simulink model "sampleModel1878"  (R2023a)
settings: Solver=VariableStepAuto  StartTime=0.0  StopTime=10.0  RelTol=1e-3
libraries: hdlsllib x5
settings Model: Creator=user1  LastModifiedBy=user1

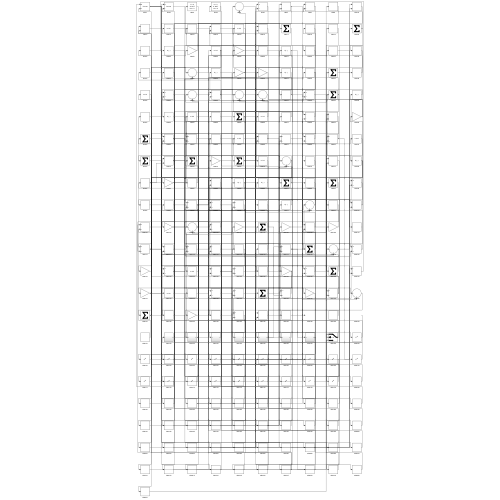
[thumbnail: Simulink's stored preview of the top-level diagram]
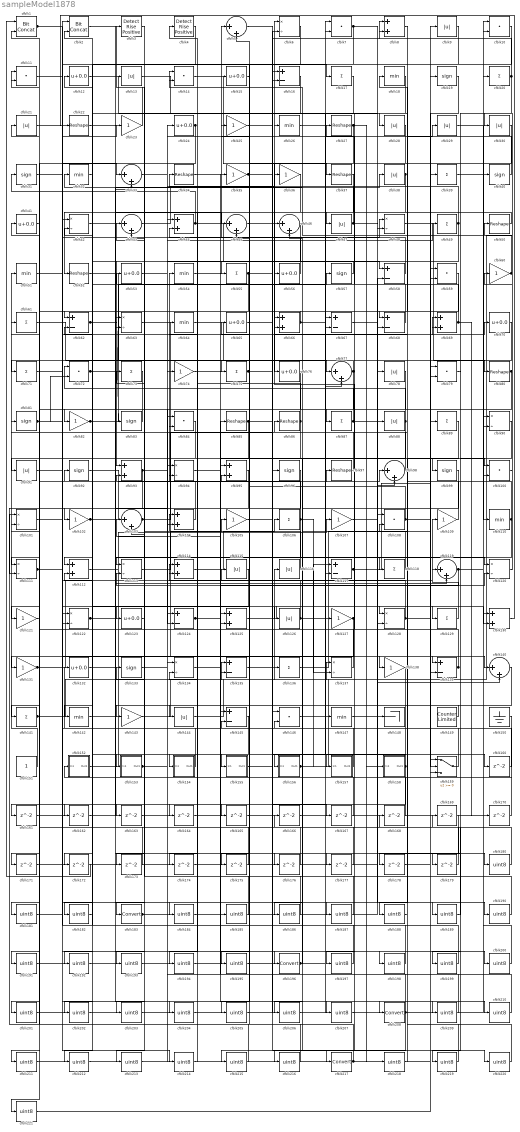
== system sampleModel1878 ==
  cfblk1 : hdlsllib/Logic and Bit Operations/Bit Concat  numInputs=2
  cfblk{7,10..11,14,59,72,79,84,100,108,146} (11 alike) : DotProduct  OutDataTypeStr=Inherit: Inherit via internal rule
  cfblk{6,42,48,63,90,94,101,111,113,120,122,128,134,137} (14 alike) : Product  Inputs=*/  RndMeth=Zero  SaturateOnIntegerOverflow=on
  cfblk{23,25,35..36,60,74,82,102,105,107,109,121,127,131,138,143} (16 alike) : Gain
  cfblk{5,33,43,45..46,77,98,103,119,140} (10 alike) : Sum  Inputs=|++
  cfblk{8,44,66,69,93,95,104,112,114,125,130} (11 alike) : Sum
  cfblk{17,20,39,49,55,61,71,73,75,87,89,106,118,129,136,141} (16 alike) : Sum  Inputs=+
  cfblk{18,26,32,51,54,64,110,142,147} (9 alike) : MinMax
  cfblk{9,13,21,28..30,38,47,78,88,91,115..116,126,144} (15 alike) : Abs  SaturateOnIntegerOverflow=off
  cfblk{16,58,62,67..68,117,124,135,139,145} (10 alike) : Sum  Inputs=+-
  cfblk{12,15,24,41,53,56,65,70,76,123,132} (11 alike) : Bias  Bias=0.0  SaturateOnIntegerOverflow=off
  cfblk{19,31,40,57,81,83,92,96,99,133} (10 alike) : Signum
  cfblk148 : Terminator
  cfblk149 : hdlsllib/Sources/Counter Limited  uplimit=7  tsamp=-1
  cfblk150 : Ground
  cfblk151 : Constant  SampleTime=-1
  cfblk152 : Subsystem
      settings: LibrarySourceBlock=|
      | hdlsllib/Ports &
      | Subsystems/Subsystem
  cfblk153 : Subsystem
      settings: LibrarySourceBlock=|
      | hdlsllib/Ports &
      | Subsystems/Subsystem
  cfblk154 : Subsystem
      settings: LibrarySourceBlock=|
      | hdlsllib/Ports &
      | Subsystems/Subsystem
  cfblk155 : Subsystem
      settings: LibrarySourceBlock=|
      | hdlsllib/Ports &
      | Subsystems/Subsystem
  cfblk156 : Subsystem
      settings: LibrarySourceBlock=|
      | hdlsllib/Ports &
      | Subsystems/Subsystem
  cfblk157 : Subsystem
      settings: LibrarySourceBlock=|
      | hdlsllib/Ports &
      | Subsystems/Subsystem
  cfblk158 : Subsystem
      settings: LibrarySourceBlock=|
      | hdlsllib/Ports &
      | Subsystems/Subsystem
  cfblk159 : Switch  SaturateOnIntegerOverflow=off  InputSameDT=off
  cfblk{160..179} (20 alike) : Delay  SampleTime=1
  cfblk{180..182,184..195,197..207,209..216,218..221} (38 alike) : DataTypeConversion  OutDataTypeStr=uint8  SaturateOnIntegerOverflow=off  RndMeth=Floor
  cfblk{183,196,208,217} (4 alike) : DataTypeConversion  SaturateOnIntegerOverflow=off  RndMeth=Floor
  cfblk2 : hdlsllib/Logic and Bit Operations/Bit Concat  numInputs=2
  cfblk{22,27,34,37,50,52,80,85..86,97} (10 alike) : Reshape
  cfblk3 : hdlsllib/Logic and Bit Operations/Detect Rise Positive  vinit=0  OutDataTypeStr=boolean
  cfblk4 : hdlsllib/Logic and Bit Operations/Detect Rise Positive  vinit=0  OutDataTypeStr=boolean
  wires:
  cfblk88/1 -> cfblk72/1, cfblk191/1, cfblk216/1
  cfblk152/1(Out1) -> cfblk107/1
  cfblk143/1 -> cfblk135/1
  cfblk139/1 -> cfblk6/1, cfblk41/1
  cfblk28/1 -> cfblk76/1
  cfblk50/1 -> cfblk47/1
  cfblk40/1 -> cfblk28/1
  cfblk68/1 -> cfblk27/1
  cfblk46/1 -> cfblk93/1
  cfblk156/1(Out1) -> cfblk30/1, cfblk117/1
  cfblk114/1 -> cfblk106/1
  cfblk92/1 -> cfblk98/1
  cfblk57/1 -> cfblk55/1
  cfblk151/1 -> cfblk51/1
  cfblk82/1 -> cfblk56/1, cfblk125/2
  cfblk39/1 -> cfblk20/1
  cfblk104/1 -> cfblk54/1
  cfblk63/1 -> cfblk135/2
  cfblk102/1 -> cfblk88/1, cfblk104/2
  cfblk110/1 -> cfblk81/1, cfblk113/1
  cfblk83/1 -> cfblk82/1
  cfblk60/1 -> cfblk32/1, cfblk14/1
  cfblk54/1 -> cfblk99/1
  cfblk38/1 -> cfblk112/1, cfblk194/1
  cfblk147/1 -> cfblk148/1
  cfblk48/1 -> cfblk80/1
  cfblk69/1 -> cfblk12/1, cfblk170/1
  cfblk106/1 -> cfblk21/1, cfblk62/2, cfblk137/2, cfblk195/1
  cfblk65/1 -> cfblk46/1
  cfblk127/1 -> cfblk181/1, cfblk206/1
  cfblk128/1 -> cfblk115/1, cfblk70/1
  cfblk18/1 -> cfblk217/1
  cfblk14/1 -> cfblk37/1
  cfblk31/1 -> cfblk23/1
  cfblk105/1 -> cfblk57/1
  cfblk121/1 -> cfblk11/1
  cfblk4/1 -> cfblk183/1
  cfblk62/1 -> cfblk83/1, cfblk119/2
  cfblk117/1 -> cfblk89/1, cfblk218/1
  cfblk136/1 -> cfblk39/1
  cfblk37/1 -> cfblk52/1
  cfblk24/1 -> cfblk141/1, cfblk121/1
  cfblk44/1 -> cfblk108/1, cfblk31/1
  cfblk120/1 -> cfblk60/1
  cfblk8/1 -> cfblk68/1
  cfblk144/1 -> cfblk116/1
  cfblk150/1 -> cfblk152/1(In1)
  cfblk98/1 -> cfblk73/1
  cfblk55/1 -> cfblk154/1(In1), cfblk117/2
  cfblk113/1 -> cfblk105/1
  cfblk23/1 -> cfblk3/1
  cfblk159/1 -> cfblk114/1
  cfblk141/1 -> cfblk61/1, cfblk9/1
  cfblk75/1 -> cfblk8/1, cfblk220/1
  cfblk131/1 -> cfblk24/1, cfblk119/1
  cfblk118/1 -> cfblk86/1
  cfblk47/1 -> cfblk34/1, cfblk140/2
  cfblk130/1 -> cfblk22/1
  cfblk43/1 -> cfblk36/1
  cfblk78/1 -> cfblk131/1
  cfblk27/1 -> cfblk158/1(In1), cfblk165/1
  cfblk124/1 -> cfblk120/2, cfblk176/1
  cfblk76/1 -> cfblk124/2
  cfblk125/1 -> cfblk128/1
  cfblk100/1 -> cfblk50/1
  cfblk153/1(Out1) -> cfblk97/1, cfblk213/1
  cfblk77/1 -> cfblk71/1, cfblk155/1(In1), cfblk161/1
  cfblk56/1 -> cfblk5/1
  cfblk97/1 -> cfblk25/1
  cfblk52/1 -> cfblk75/1
  cfblk123/1 -> cfblk103/2
  cfblk126/1 -> cfblk19/1, cfblk104/1
  cfblk42/1 -> cfblk196/1
  cfblk61/1 -> cfblk77/1
  cfblk81/1 -> cfblk126/1, cfblk72/2
  cfblk7/1 -> cfblk68/2, cfblk142/1
  cfblk19/1 -> cfblk159/2
  cfblk70/1 -> cfblk87/1
  cfblk133/1 -> cfblk35/1
  cfblk86/1 -> cfblk64/1, cfblk192/1
  cfblk140/1 -> cfblk156/1(In1)
  cfblk129/1 -> cfblk109/1
  cfblk154/1(Out1) -> cfblk132/1
  cfblk137/1 -> cfblk5/2
  cfblk103/1 -> cfblk6/2, cfblk53/1
  cfblk45/1 -> cfblk96/1
  cfblk51/1 -> cfblk138/1
  cfblk64/1 -> cfblk147/1
  cfblk49/1 -> cfblk102/1, cfblk14/2
  cfblk11/1 -> cfblk17/1
  cfblk41/1 -> cfblk111/1
  cfblk26/1 -> cfblk77/2
  cfblk111/1 -> cfblk48/1, cfblk184/1
  cfblk155/1(Out1) -> cfblk137/1
  cfblk58/1 -> cfblk44/2
  cfblk72/1 -> cfblk118/1, cfblk66/2
  cfblk53/1 -> cfblk58/1
  cfblk108/1 -> cfblk65/1, cfblk140/1
  cfblk3/1 -> cfblk63/1
  cfblk12/1 -> cfblk127/1
  cfblk96/1 -> cfblk122/2
  cfblk20/1 -> cfblk8/2, cfblk179/1
  cfblk21/1 -> cfblk130/2
  cfblk157/1(Out1) -> cfblk43/2
  cfblk87/1 -> cfblk13/1, cfblk120/1
  cfblk29/1 -> cfblk110/1
  cfblk85/1 -> cfblk123/1, cfblk100/1
  cfblk149/1 -> cfblk143/1
  cfblk74/1 -> cfblk129/1
  cfblk116/1 -> cfblk92/1
  cfblk33/1 -> cfblk29/1
  cfblk122/1 -> cfblk38/1, cfblk139/2
  cfblk94/1 -> cfblk208/1
  cfblk17/1 -> cfblk63/2
  cfblk109/1 -> cfblk66/1
  cfblk80/1 -> cfblk91/1, cfblk144/1, cfblk163/1
  cfblk66/1 -> cfblk62/1, cfblk100/2
  cfblk35/1 -> cfblk157/1(In1), cfblk15/1
  cfblk112/1 -> cfblk85/1
  cfblk119/1 -> cfblk40/1, cfblk113/2
  cfblk93/1 -> cfblk26/1, cfblk111/2, cfblk49/1
  cfblk91/1 -> cfblk69/1
  cfblk22/1 -> cfblk45/1
  cfblk1/1 -> cfblk33/1, cfblk139/1, cfblk198/1, cfblk207/1
  cfblk107/1 -> cfblk69/2
  cfblk158/1(Out1) -> cfblk153/1(In1), cfblk201/1, cfblk221/1
  cfblk13/1 -> cfblk48/2
  cfblk146/1 -> cfblk160/1
  cfblk160/1 -> cfblk122/1
  cfblk161/1 -> cfblk33/2
  cfblk115/1 -> cfblk162/1
  cfblk163/1 -> cfblk58/2
  cfblk145/1 -> cfblk164/1
  cfblk164/1 -> cfblk128/2
  cfblk165/1 -> cfblk159/1
  cfblk166/1 -> cfblk130/1
  cfblk25/1 -> cfblk167/1
  cfblk167/1 -> cfblk112/2
  cfblk168/1 -> cfblk45/2
  cfblk170/1 -> cfblk46/2
  cfblk73/1 -> cfblk171/1
  cfblk171/1 -> cfblk98/2
  cfblk32/1 -> cfblk172/1
  cfblk172/1 -> cfblk1/1
  cfblk9/1 -> cfblk173/1
  cfblk173/1 -> cfblk1/2
  cfblk36/1 -> cfblk174/1
  cfblk174/1 -> cfblk114/2
  cfblk15/1 -> cfblk175/1
  cfblk175/1 -> cfblk11/2
  cfblk176/1 -> cfblk44/1
  cfblk132/1 -> cfblk177/1
  cfblk177/1 -> cfblk103/1
  cfblk89/1 -> cfblk178/1
  cfblk178/1 -> cfblk159/3
  cfblk179/1 -> cfblk93/2
  cfblk2/1 -> cfblk180/1
  cfblk180/1 -> cfblk145/1
  cfblk181/1 -> cfblk2/1
  cfblk138/1 -> cfblk182/1
  cfblk182/1 -> cfblk2/2
  cfblk183/1 -> cfblk136/1, cfblk78/1
  cfblk184/1 -> cfblk4/1
  cfblk134/1 -> cfblk185/1
  cfblk185/1 -> cfblk133/1
  cfblk99/1 -> cfblk186/1
  cfblk186/1 -> cfblk134/1
  cfblk135/1 -> cfblk187/1
  cfblk187/1 -> cfblk134/2
  cfblk169/1 -> cfblk188/1
  cfblk188/1 -> cfblk108/2
  cfblk142/1 -> cfblk189/1
  cfblk189/1 -> cfblk169/1
  cfblk67/1 -> cfblk190/1
  cfblk190/1 -> cfblk43/1
  cfblk191/1 -> cfblk67/1
  cfblk192/1 -> cfblk67/2
  cfblk95/1 -> cfblk193/1
  cfblk193/1 -> cfblk74/1
  cfblk194/1 -> cfblk95/1
  cfblk195/1 -> cfblk95/2
  cfblk196/1 -> cfblk7/2, cfblk146/2
  cfblk30/1 -> cfblk197/1
  cfblk197/1 -> cfblk42/1
  cfblk198/1 -> cfblk42/2
  cfblk90/1 -> cfblk199/1
  cfblk199/1 -> cfblk166/1
  cfblk34/1 -> cfblk200/1
  cfblk200/1 -> cfblk90/1
  cfblk201/1 -> cfblk90/2
  cfblk16/1 -> cfblk202/1
  cfblk202/1 -> cfblk146/1
  cfblk84/1 -> cfblk203/1
  cfblk203/1 -> cfblk16/1
  cfblk71/1 -> cfblk204/1
  cfblk204/1 -> cfblk16/2
  cfblk10/1 -> cfblk205/1
  cfblk205/1 -> cfblk7/1
  cfblk206/1 -> cfblk10/1
  cfblk207/1 -> cfblk10/2
  cfblk208/1 -> cfblk125/1, cfblk215/1
  cfblk162/1 -> cfblk209/1
  cfblk209/1 -> cfblk94/1
  cfblk5/1 -> cfblk210/1
  cfblk210/1 -> cfblk94/2
  cfblk59/1 -> cfblk211/1
  cfblk211/1 -> cfblk84/1
  cfblk6/1 -> cfblk212/1
  cfblk212/1 -> cfblk59/1
  cfblk213/1 -> cfblk59/2
  cfblk101/1 -> cfblk214/1
  cfblk214/1 -> cfblk84/2
  cfblk215/1 -> cfblk101/1
  cfblk216/1 -> cfblk101/2
  cfblk217/1 -> cfblk145/2, cfblk124/1
  cfblk218/1 -> cfblk18/1
  cfblk79/1 -> cfblk219/1
  cfblk219/1 -> cfblk168/1
  cfblk220/1 -> cfblk79/1
  cfblk221/1 -> cfblk79/2

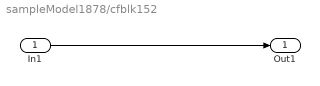
== system sampleModel1878/cfblk152 ==
  In1 : Inport
  Out1 : Outport
  wires:
  In1/1 -> Out1/1

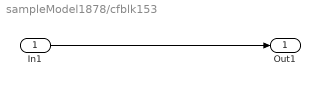
== system sampleModel1878/cfblk153 ==
  In1 : Inport
  Out1 : Outport
  wires:
  In1/1 -> Out1/1

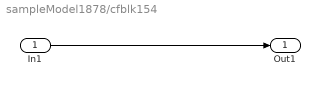
== system sampleModel1878/cfblk154 ==
  In1 : Inport
  Out1 : Outport
  wires:
  In1/1 -> Out1/1

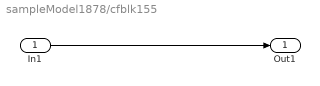
== system sampleModel1878/cfblk155 ==
  In1 : Inport
  Out1 : Outport
  wires:
  In1/1 -> Out1/1

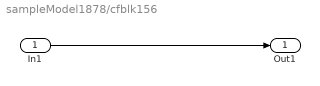
== system sampleModel1878/cfblk156 ==
  In1 : Inport
  Out1 : Outport
  wires:
  In1/1 -> Out1/1

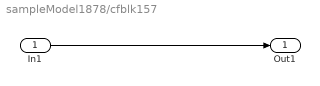
== system sampleModel1878/cfblk157 ==
  In1 : Inport
  Out1 : Outport
  wires:
  In1/1 -> Out1/1

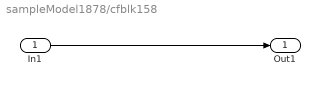
== system sampleModel1878/cfblk158 ==
  In1 : Inport
  Out1 : Outport
  wires:
  In1/1 -> Out1/1
